simulink model "SixStep_Commutation_dsPIC33CK_Curiosity"  (R2023a)
settings: Solver=FixedStepDiscrete  StartTime=0.0  StopTime=10.0  FixedStep=50e-6  RelTol=1e-3  EnableMultiTasking=on
undefined symbols (not defined in the file): MaxPer, PWM1max, Resol, s, us
libraries: MCHP_Blockset x18, simulink x5
(part 2 of 2)

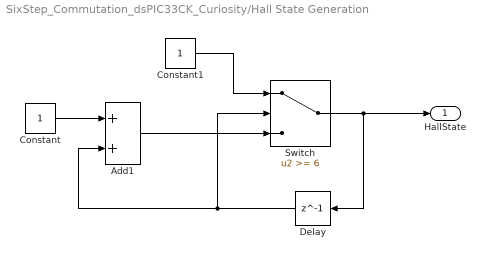
== system SixStep_Commutation_dsPIC33CK_Curiosity/Hall State Generation ==
  Add1 : Sum  SaturateOnIntegerOverflow=on
  Constant : Constant  OutDataTypeStr=uint16  SampleTime=0.2e-3
  Constant1 : Constant  OutDataTypeStr=uint16  SampleTime=0.2e-3
  Delay : Delay  DelayLength=1
  Switch : Switch  Threshold=6  SaturateOnIntegerOverflow=off  InputSameDT=off
  HallState : Outport
  wires:
  Delay/1 -> Add1/2, Switch/2
  Switch/1 -> HallState/1, Delay/1
  Add1/1 -> Switch/3
  Constant/1 -> Add1/1
  Constant1/1 -> Switch/1

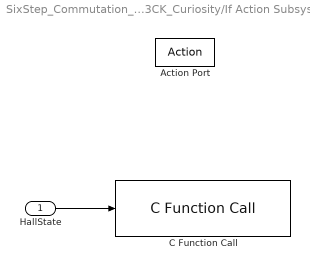
== system SixStep_Commutation_dsPIC33CK_Curiosity/If Action Subsystem ==
  HallState : Inport
  Action Port : ActionPort  ActionPortLabel=if(u1 == 0)
  C Function Call : MCHP_Blockset/User Functions/C Function Call  ParseFilesChkbx=on  ListFunctions1=Custom Function  Function1=void PWMOverride_Scheme1(unsigned int sector)  AddHeaderDeclaration=on  Function1Type=when block is updated (default)  Fct1BlockIn=sector  FctReturnBlockOut=on  DataCollected=s.chksm={ '242523-May-2023 09:29:41'};s.File1={};  ORDERING=None  SampleTime=-1  S_INPUT=0  S_INPUT_Size=0  S_OUTPUT=0  S_OUTPUT_Size=0  S_ListCustomDatatype=0  MCHP_CRC=1056480  MCHP_MASTERLINK=SixStep_Commutation_dsPIC33CK_Curiosity/Curiosity Board/Microchip Master  PinDigitalInput=[]  PinDigitalOutput=[]  PinAnalogInput=[]
      settings: SourceProductName=MPLAB Device Blocks for Simulink
  wires:
  HallState/1 -> C Function Call/1

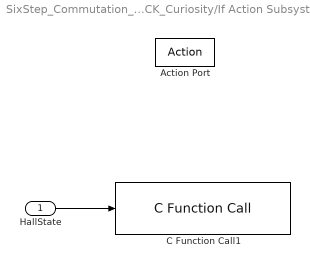
== system SixStep_Commutation_dsPIC33CK_Curiosity/If Action Subsystem1 ==
  HallState : Inport
  Action Port : ActionPort  ActionPortLabel=elseif(u1 == 1)
  C Function Call1 : MCHP_Blockset/User Functions/C Function Call  ParseFilesChkbx=on  ListFunctions1=Custom Function  Function1=void PWMOverride_Scheme2(unsigned int sector)  AddHeaderDeclaration=on  Function1Type=when block is updated (default)  Fct1BlockIn=sector  FctReturnBlockOut=on  DataCollected=s.chksm={ '150615-May-2023 17:09:02'};s.File1={};  ORDERING=None  SampleTime=-1  S_INPUT=0  S_INPUT_Size=0  S_OUTPUT=0  S_OUTPUT_Size=0  S_ListCustomDatatype=0  MCHP_CRC=1056342  MCHP_MASTERLINK=SixStep_Commutation_dsPIC33CK_Curiosity/Curiosity Board/Microchip Master  PinDigitalInput=[]  PinDigitalOutput=[]  PinAnalogInput=[]
      settings: SourceProductName=MPLAB Device Blocks for Simulink
  wires:
  HallState/1 -> C Function Call1/1

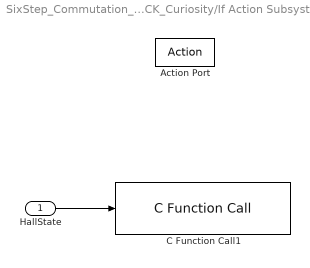
== system SixStep_Commutation_dsPIC33CK_Curiosity/If Action Subsystem2 ==
  HallState : Inport
  Action Port : ActionPort  ActionPortLabel=else
  C Function Call1 : MCHP_Blockset/User Functions/C Function Call  ParseFilesChkbx=on  ListFunctions1=Custom Function  Function1=void PWMOverride_Scheme3(unsigned int sector)  AddHeaderDeclaration=on  Function1Type=when block is updated (default)  Fct1BlockIn=sector  FctReturnBlockOut=on  DataCollected=s.chksm={ '150615-May-2023 17:09:02'};s.File1={};  ORDERING=None  SampleTime=-1  S_INPUT=0  S_INPUT_Size=0  S_OUTPUT=0  S_OUTPUT_Size=0  S_ListCustomDatatype=0  MCHP_CRC=1056473  MCHP_MASTERLINK=SixStep_Commutation_dsPIC33CK_Curiosity/Curiosity Board/Microchip Master  PinDigitalInput=[]  PinDigitalOutput=[]  PinAnalogInput=[]
      settings: SourceProductName=MPLAB Device Blocks for Simulink
  wires:
  HallState/1 -> C Function Call1/1

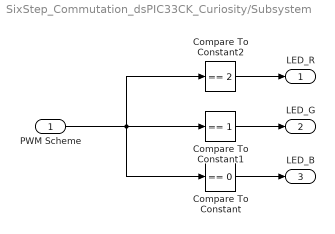
== system SixStep_Commutation_dsPIC33CK_Curiosity/Subsystem ==
  PWM Scheme : Inport
  Compare To Constant : simulink/Logic and Bit Operations/Compare To Constant  relop===  const=0  OutDataTypeStr=boolean
  Compare To Constant1 : simulink/Logic and Bit Operations/Compare To Constant  relop===  const=1  OutDataTypeStr=boolean
  Compare To Constant2 : simulink/Logic and Bit Operations/Compare To Constant  relop===  const=2  OutDataTypeStr=boolean
  LED_R : Outport
  LED_G : Outport  Port=2
  LED_B : Outport  Port=3
  wires:
  Compare To Constant/1 -> LED_B/1
  PWM Scheme/1 -> Compare To Constant/1, Compare To Constant2/1, Compare To Constant1/1
  Compare To Constant1/1 -> LED_G/1
  Compare To Constant2/1 -> LED_R/1

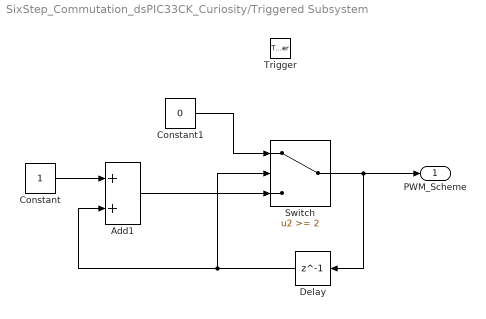
== system SixStep_Commutation_dsPIC33CK_Curiosity/Triggered Subsystem ==
  Trigger : TriggerPort  TriggerType=falling  VariantControl=Variant
  Add1 : Sum  SaturateOnIntegerOverflow=on
  Constant : Constant  OutDataTypeStr=uint16
  Constant1 : Constant  Value=0  OutDataTypeStr=uint16
  Delay : Delay  DelayLength=1
  Switch : Switch  Threshold=2  SaturateOnIntegerOverflow=off  InputSameDT=off
  PWM_Scheme : Outport
  wires:
  Constant/1 -> Add1/1
  Delay/1 -> Add1/2, Switch/2
  Add1/1 -> Switch/3
  Switch/1 -> Delay/1, PWM_Scheme/1
  Constant1/1 -> Switch/1

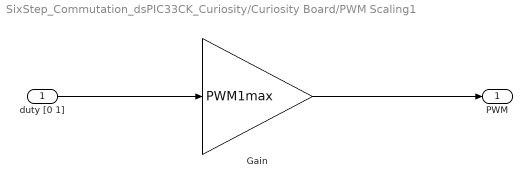
== system SixStep_Commutation_dsPIC33CK_Curiosity/Curiosity Board/PWM Scaling1 ==
  duty [0 1] : Inport
  Gain : Gain  Gain=PWM1max  OutDataTypeStr=uint16
  PWM : Outport  VectorParamsAs1DForOutWhenUnconnected=off
  wires:
  duty [0 1]/1 -> Gain/1
  Gain/1 -> PWM/1
